simulink model "barra1"  (R2020a)
settings: Solver=ode45  StartTime=0.0  StopTime=tfinal  RelTol=1e-6  EnableMultiTasking=on
values from neighbouring files (symbols this model uses):
  Atrue = [-4496779.27487 -22483886.9993 -13490335.5746 -17987111.287 -4496779.27487 -2248391.44993 -4974615.90913 -24873081.1934 -14923848.4319 -19898464.4945 -4974616.00004 -2487308.09661 ... (36 elements, 6x6)]    [barrassmodel.mat]
  Btrue = [1 5 3 4 1 0.5]    [barrassmodel.mat]
  Ctrue = [26671680 -23900596.3636 330105338.182 -153564218.182 -183930676.364 -198594327.273]    [barrassmodel.mat]
  Dtrue = 0    [barrassmodel.mat]
  Ts = 1/fs    (= 0.001)    [BasicSim.m]    (also in IdentificationAlgorithm_best.m = 0.01)
undefined symbols (not defined in the file or in its folder): flag
settings Model: Creator=jomle  LastModifiedBy=renato
settings DataIOCC: LimitDataPoints=on  SaveFormat=Array  ReturnWorkspaceOutputs=off
settings OptimizationCC: LifeSpan=inf
settings DebuggingCC: SFUnexpectedBacktrackingDiag=warning  SFNoUnconditionalDefaultTransitionDiag=warning  SFExecutionAtInitializationDiag=none  ArithmeticOperatorsInVariantConditions=warning
settings HardwareCC: ProdBitPerPointer=32  ProdBitPerSizeT=32  ProdBitPerPtrDiffT=32  ProdLargestAtomicFloat=None  ProdIntDivRoundTo=Undefined  ProdEndianess=Unspecified  ProdWordSize=32  ProdHWDeviceType=32-bit Generic
settings ModelReferenceCC: PropagateSignalLabelsOutOfModel=off
settings SFSimCC: SimUseLocalCustomCode=off  CustomCodeUndefinedFunction=UseInterfaceOnly
settings RTWCC: RTWUseLocalCustomCode=off
settings CodeAppCC: StateflowObjectComments=on
settings GRTTargetCC: TargetLangStandard=C89/C90 (ANSI)
settings ConfigComp: CovMetricSettings=dw  CovHtmlReporting=on  CovSaveCumulativeToWorkspaceVar=on  CovSaveSingleToWorkspaceVar=on  CovExternalEMLEnable=off

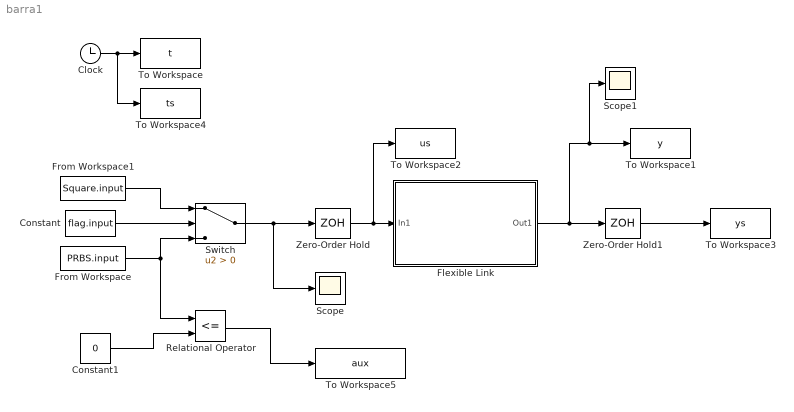
== system barra1 ==
  Clock : Clock
  Constant : Constant  Value=flag.input
  Constant1 : Constant  Value=0
  Flexible Link : Subsystem
      mask Display: image('quanserlink.jpg')
  From Workspace : FromWorkspace  VariableName=PRBS.input
  From Workspace1 : FromWorkspace  VariableName=Square.input
  Relational Operator : RelationalOperator  Operator=<=  OutDataTypeStr=boolean  RndMeth=Simplest
  Scope : Scope
  Scope1 : Scope
  Switch : Switch  Criteria=u2 > Threshold
  To Workspace : ToWorkspace  VariableName=t  SampleTime=-1
  To Workspace1 : ToWorkspace  VariableName=y  SampleTime=-1
  To Workspace2 : ToWorkspace  VariableName=us  SampleTime=Ts
  To Workspace3 : ToWorkspace  VariableName=ys  SampleTime=Ts
  To Workspace4 : ToWorkspace  VariableName=ts  SampleTime=Ts
  To Workspace5 : ToWorkspace  VariableName=aux  SaveFormat=Timeseries  SampleTime=-1
  Zero-Order Hold : ZeroOrderHold  SampleTime=Ts
  Zero-Order Hold1 : ZeroOrderHold  SampleTime=Ts
  wires:
  Clock/1 -> To Workspace4/1, To Workspace/1
  Zero-Order Hold/1 -> To Workspace2/1, Flexible Link/1(In1)
  Flexible Link/1(Out1) -> Scope1/1, To Workspace1/1, Zero-Order Hold1/1
  Zero-Order Hold1/1 -> To Workspace3/1
  From Workspace/1 -> Relational Operator/1, Switch/3
  Constant/1 -> Switch/2
  From Workspace1/1 -> Switch/1
  Constant1/1 -> Relational Operator/2
  Relational Operator/1 -> To Workspace5/1
  Switch/1 -> Scope/1, Zero-Order Hold/1

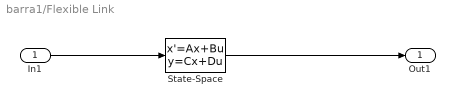
== system barra1/Flexible Link ==
  In1 : Inport
  State-Space : StateSpace  A=Atrue  B=Btrue  C=Ctrue  D=Dtrue  InitialCondition=0
  Out1 : Outport
  wires:
  State-Space/1 -> Out1/1
  In1/1 -> State-Space/1
